simulink model "c_station_v3"  (R2019a)
settings: Solver=VariableStepAuto  StartTime=0.0  StopTime=345600  MaxStep=3600  RelTol=1e-3  AbsTol=1e-3  EnableMultiTasking=on
StopFcn:
  | displayGasParameters(gasPressures);
values from neighbouring files (symbols this model uses):
  conf = gasConfig()    [ColoradoGasModel.m]    (also in gas_v1.m)
  lineParm = [lineParm;add_line("Main 2",24,35,pNom)]    [compressorTest.m]    (also in experiment1.m = [lineParm;add_line("Main 2",24,50,pNom)]; experiment2.m = [lineParm;add_line("Main 3",24,35,pNom)]; experiment3.m = [lineParm;add_line("Aux 3",36,100,pNom)]; experiments12.m)
  loadControlFlag = "on"    [gas_v1.m]
  loadParm = [loadParm; add_load("PP2",pwr,pNom,pCut, stopTime)]    [compressorTest.m]    (also in experiment1.m; experiment2.m; experiment3.m = [loadParm; add_load("PP2",pwr,pNom,pCut,stopTime)]; experiments12.m)
  valveControlFlag = "on"    [ColoradoGasModel.m]    (also in gas_v1.m)
undefined symbols (not defined in the file or in its folder): f, valveParm
libraries: gasLibrary x27, fl_lib x14, nesl_utility x9, instrumentlib x4, SimscapeFluids_lib x1
(part 3 of 3)

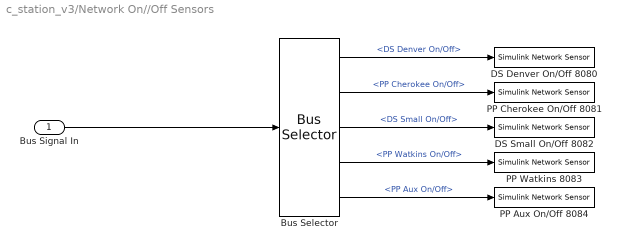
== system c_station_v3/Network On//Off Sensors ==
  Bus Signal In : Inport
  Bus Selector : BusSelector  OutputSignals=DS Denver On/Off,PP Cherokee On/Off,DS Small On/Off,PP Watkins On/Off,PP Aux On/Off
  DS Denver On/Off 8080 : gasLibrary/Simulink Network Sensor  Port=8080
  DS Small On/Off 8082 : gasLibrary/Simulink Network Sensor  Port=8082
  PP Aux On/Off 8084 : gasLibrary/Simulink Network Sensor  Port=8084
  PP Cherokee On/Off 8081 : gasLibrary/Simulink Network Sensor  Port=8081
  PP Watkins 8083 : gasLibrary/Simulink Network Sensor  Port=8083
  wires:
  Bus Selector/1 -> DS Denver On/Off 8080/1  "<DS Denver On/Off>"
  Bus Signal In/1 -> Bus Selector/1
  Bus Selector/2 -> PP Cherokee On/Off 8081/1  "<PP Cherokee On/Off>"
  Bus Selector/4 -> PP Watkins 8083/1  "<PP Watkins On/Off>"
  Bus Selector/5 -> PP Aux On/Off 8084/1  "<PP Aux On/Off>"
  Bus Selector/3 -> DS Small On/Off 8082/1  "<DS Small On/Off>"

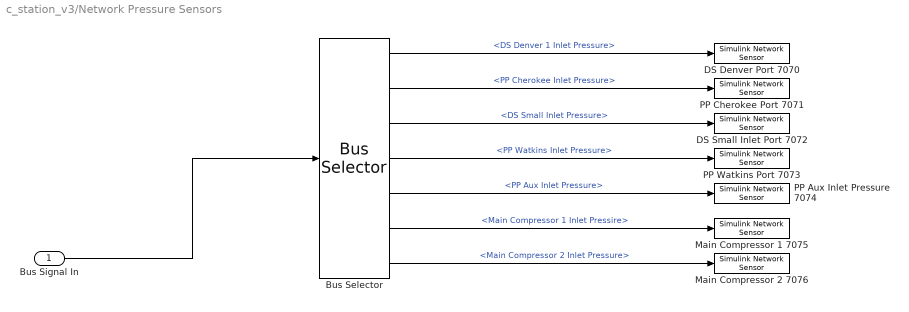
== system c_station_v3/Network Pressure Sensors ==
  Bus Signal In : Inport
  Bus Selector : BusSelector  OutputSignals=DS Denver 1 Inlet Pressure,PP Cherokee Inlet Pressure,DS Small Inlet Pressure,PP Watkins Inlet Pressure,PP Aux Inlet Pressure,Main Compressor 1 Inlet Pressire,Main Compressor 2 Inlet Pressure
  DS Denver Port 7070 : gasLibrary/Simulink Network Sensor  Port=7070
  DS Small Inlet Port 7072 : gasLibrary/Simulink Network Sensor  Port=7072
  Main Compressor 1 7075 : gasLibrary/Simulink Network Sensor  Port=7075
  Main Compressor 2 7076 : gasLibrary/Simulink Network Sensor  Port=7076
  PP Aux Inlet Pressure 7074 : gasLibrary/Simulink Network Sensor  Port=7074
  PP Cherokee Port 7071 : gasLibrary/Simulink Network Sensor  Port=7071
  PP Watkins Port 7073 : gasLibrary/Simulink Network Sensor  Port=7073
  wires:
  Bus Selector/4 -> PP Watkins Port 7073/1  "<PP Watkins Inlet Pressure>"
  Bus Signal In/1 -> Bus Selector/1
  Bus Selector/2 -> PP Cherokee Port 7071/1  "<PP Cherokee Inlet Pressure>"
  Bus Selector/3 -> DS Small Inlet Port 7072/1  "<DS Small Inlet Pressure>"
  Bus Selector/1 -> DS Denver Port 7070/1  "<DS Denver 1 Inlet Pressure>"
  Bus Selector/6 -> Main Compressor 1 7075/1  "<Main Compressor 1 Inlet Pressire>"
  Bus Selector/7 -> Main Compressor 2 7076/1  "<Main Compressor 2 Inlet Pressure>"
  Bus Selector/5 -> PP Aux Inlet Pressure 7074/1  "<PP Aux Inlet Pressure>"

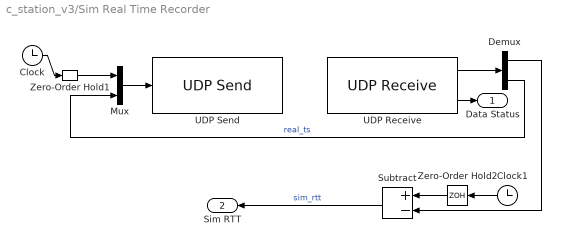
== system c_station_v3/Sim Real Time Recorder ==
  Clock : Clock
  Clock1 : Clock
  Demux : Demux  Outputs=2
  Mux : Mux  Inputs=2
  Subtract : Sum  Inputs=+-
  UDP Receive : instrumentlib/UDP Receive  Priority=2  Host=localhost  Port=5001  LocalPort=6065  EnablePortSharing=off  GetLatestData=off  DataSize="[2  1]"  DataType=double  ASCIIFormatting=%f,  Terminator=LF  ByteOrder=BigEndian  EnableBlockingMode=off  Timeout=50  SampleTime=60  LocalAddress=localhost
      settings: SourceProductName=Instrument Control Toolbox
  UDP Send : instrumentlib/UDP Send  Priority=1  Host=localhost  Port=6068  LocalPort=-1  EnablePortSharing=off  ByteOrder=BigEndian  OutputDatagramPacketSize=24  EnableBlockingMode=on  LocalAddress=0.0.0.0
      settings: SourceProductName=Instrument Control Toolbox
  Zero-Order Hold1 : ZeroOrderHold  SampleTime=60
  Zero-Order Hold2 : ZeroOrderHold  SampleTime=60
  Data Status : Outport
  Sim RTT : Outport  Port=2
  wires:
  Clock1/1 -> Zero-Order Hold2/1
  Clock/1 -> Zero-Order Hold1/1
  Demux/1 -> Subtract/2
  UDP Receive/1 -> Demux/1
  Demux/2 -> Mux/2  "real_ts"
  UDP Receive/2 -> Data Status/1
  Mux/1 -> UDP Send/1
  Zero-Order Hold2/1 -> Subtract/1
  Zero-Order Hold1/1 -> Mux/1
  Subtract/1 -> Sim RTT/1  "sim_rtt"

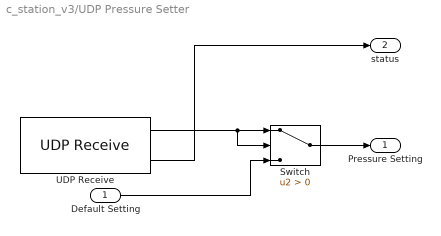
== system c_station_v3/UDP Pressure Setter ==
  Default Setting : Inport
  Switch : Switch  Criteria=u2 > Threshold
  UDP Receive : instrumentlib/UDP Receive  Host=localhost  Port=5000  LocalPort=LocalPort  EnablePortSharing=off  GetLatestData=on  DataSize=[1 1]  DataType=double  ASCIIFormatting=%f,  Terminator=LF  ByteOrder=BigEndian  EnableBlockingMode=off  Timeout=10  SampleTime=300  LocalAddress=localhost
      settings: SourceProductName=Instrument Control Toolbox
  "Pressure Setting " : Outport
  status : Outport  Port=2
  wires:
  UDP Receive/2 -> status/1
  UDP Receive/1 -> Switch/1, Switch/2
  Switch/1 -> "Pressure Setting "/1
  Default Setting/1 -> Switch/3

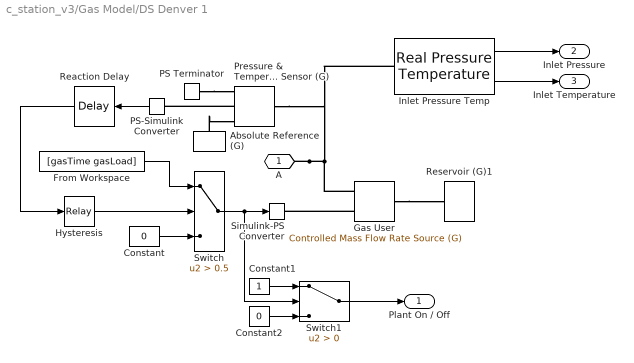
== system c_station_v3/Gas Model/DS Denver 1 ==
  Absolute Reference (G) : fl_lib/Gas/Elements/Absolute Reference (G)
      settings: SourceProductName=Simscape  SourceProductBaseCode=SS
  Constant : Constant  Value=0
  Constant1 : Constant
  Constant2 : Constant  Value=0
  From Workspace : FromWorkspace  VariableName=[gasTime gasLoad]  SampleTime=0  OutputAfterFinalValue=Holding final value
  Gas User : fl_lib/Gas/Sources/Controlled Mass Flow Rate Source (G)  power_spec=1  area_A=24^2*pi/4 in^2  area_B=20^2*pi/4 in^2  mdot_A_specify=on  mdot_A_priority=None  mdot_A=20 kg/s  mdot_A_nominal_specify=off  mdot_A_nominal_unit=kg/s  mdot_A_nominal_value=1
      settings: SourceProductName=Simscape  SourceProductBaseCode=SS
  Hysteresis : Relay  OnSwitchValue=pCutoff*1.05  OffSwitchValue=pCutoff
  Inlet Pressure Temp : gasLibrary/Real Pressure Temperature  SystemSampleTime=-1
  PS Terminator : fl_lib/Physical Signals/Sinks/PS Terminator
      settings: SourceProductName=Simscape
  PS-Simulink Converter : nesl_utility/PS-Simulink Converter  PhysicalDomain=network_engine_domain  SubClassName=ps_output  LeftPortType=input  RightPortType=output  PseudoPeriodic=off  Frequencies=[]  Unit=psi  AffineConversion=off
  Pressure & Temperature Sensor (G) : fl_lib/Gas/Sensors/Pressure & Temperature Sensor (G)
      settings: SourceProductName=Simscape  SourceProductBaseCode=SS
  Reaction Delay : TransportDelay  DelayTime=60  InitialOutput=pNominal
  Reservoir (G)1 : fl_lib/Gas/Elements/Reservoir (G)  pressure_spec=2  reservoir_pressure=300 psi  reservoir_temperature=25 degC  area_A=pi*25^2/4 in^2
      settings: SourceProductName=Foundation Library
  Simulink-PS Converter : nesl_utility/Simulink-PS Converter  PhysicalDomain=network_engine_domain  SubClassName=ps_input  LeftPortType=input  RightPortType=output  PseudoPeriodic=off  Frequencies=[]  NoiseDistribution=none  NoiseParameters=[]  Unit=1  AffineConversion=off  FilteringAndDerivatives=provide  SimscapeFilterOrder=1  InputFilterTimeConstant=0.001  UdotUserProvided=0
  Switch : Switch  Criteria=u2 > Threshold  Threshold=0.5
  Switch1 : Switch  Criteria=u2 > Threshold
  A : PMIOPort  Side=Left
  Plant On / Off : Outport
  Inlet Pressure : Outport  Port=2
  Inlet Temperature : Outport  Port=3
  wires:
  Inlet Pressure Temp/2 -> Inlet Temperature/1
  Inlet Pressure Temp/1 -> Inlet Pressure/1
  Constant1/1 -> Switch1/1
  Switch1/1 -> Plant On / Off/1
  Constant2/1 -> Switch1/3
  Switch/1 -> Simulink-PS Converter/1, Switch1/2
  Hysteresis/1 -> Switch/2
  Constant/1 -> Switch/3
  PS-Simulink Converter/1 -> Reaction Delay/1
  Reaction Delay/1 -> Hysteresis/1
  From Workspace/1 -> Switch/1
  connections:
  Pressure & Temperature Sensor (G)/RConn2 -- PS-Simulink Converter/LConn1
  Absolute Reference (G)/LConn1 -- Pressure & Temperature Sensor (G)/RConn1
  PS Terminator/LConn1 -- Pressure & Temperature Sensor (G)/RConn3
  Gas User/LConn2 -- Simulink-PS Converter/RConn1
  A/RConn1 -- Pressure & Temperature Sensor (G)/LConn1 -- Inlet Pressure Temp/LConn1 -- Gas User/LConn1
  Gas User/RConn1 -- Reservoir (G)1/LConn1

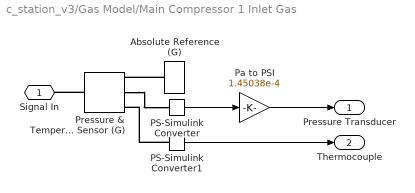
== system c_station_v3/Gas Model/Main Compressor 1 Inlet Gas ==
  Absolute Reference (G) : fl_lib/Gas/Elements/Absolute Reference (G)
      settings: SourceProductName=Simscape  SourceProductBaseCode=SS
  PS-Simulink Converter : nesl_utility/PS-Simulink Converter  PhysicalDomain=network_engine_domain  SubClassName=ps_output  LeftPortType=input  RightPortType=output  PseudoPeriodic=off  Frequencies=[]  Unit=1  AffineConversion=off
  PS-Simulink Converter1 : nesl_utility/PS-Simulink Converter  PhysicalDomain=network_engine_domain  SubClassName=ps_output  LeftPortType=input  RightPortType=output  PseudoPeriodic=off  Frequencies=[]  Unit=1  AffineConversion=off
  Pa to PSI : Gain  Gain=1.45038e-4
  Pressure & Temperature Sensor (G) : fl_lib/Gas/Sensors/Pressure & Temperature Sensor (G)
      settings: SourceProductName=Simscape  SourceProductBaseCode=SS
  Signal In : PMIOPort  Side=Left
  Pressure Transducer : Outport
  Thermocouple : Outport  Port=2
  wires:
  PS-Simulink Converter/1 -> Pa to PSI/1
  PS-Simulink Converter1/1 -> Thermocouple/1
  Pa to PSI/1 -> Pressure Transducer/1
  connections:
  Pressure & Temperature Sensor (G)/LConn1 -- Signal In/RConn1
  Absolute Reference (G)/LConn1 -- Pressure & Temperature Sensor (G)/RConn1
  PS-Simulink Converter1/LConn1 -- Pressure & Temperature Sensor (G)/RConn3
  Pressure & Temperature Sensor (G)/RConn2 -- PS-Simulink Converter/LConn1

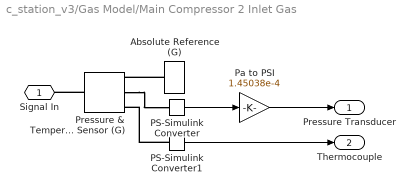
== system c_station_v3/Gas Model/Main Compressor 2 Inlet Gas ==
  Absolute Reference (G) : fl_lib/Gas/Elements/Absolute Reference (G)
      settings: SourceProductName=Simscape  SourceProductBaseCode=SS
  PS-Simulink Converter : nesl_utility/PS-Simulink Converter  PhysicalDomain=network_engine_domain  SubClassName=ps_output  LeftPortType=input  RightPortType=output  PseudoPeriodic=off  Frequencies=[]  Unit=1  AffineConversion=off
  PS-Simulink Converter1 : nesl_utility/PS-Simulink Converter  PhysicalDomain=network_engine_domain  SubClassName=ps_output  LeftPortType=input  RightPortType=output  PseudoPeriodic=off  Frequencies=[]  Unit=1  AffineConversion=off
  Pa to PSI : Gain  Gain=1.45038e-4
  Pressure & Temperature Sensor (G) : fl_lib/Gas/Sensors/Pressure & Temperature Sensor (G)
      settings: SourceProductName=Simscape  SourceProductBaseCode=SS
  Signal In : PMIOPort  Side=Left
  Pressure Transducer : Outport
  Thermocouple : Outport  Port=2
  wires:
  PS-Simulink Converter/1 -> Pa to PSI/1
  PS-Simulink Converter1/1 -> Thermocouple/1
  Pa to PSI/1 -> Pressure Transducer/1
  connections:
  Pressure & Temperature Sensor (G)/LConn1 -- Signal In/RConn1
  Absolute Reference (G)/LConn1 -- Pressure & Temperature Sensor (G)/RConn1
  PS-Simulink Converter1/LConn1 -- Pressure & Temperature Sensor (G)/RConn3
  Pressure & Temperature Sensor (G)/RConn2 -- PS-Simulink Converter/LConn1

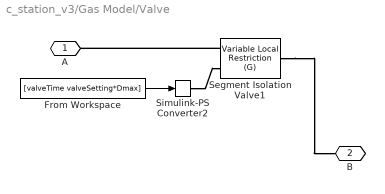
== system c_station_v3/Gas Model/Valve ==
  From Workspace : FromWorkspace  VariableName=[valveTime valveSetting*Dmax]  SampleTime=0  OutputAfterFinalValue=Holding final value
  Segment Isolation Valve1 : fl_lib/Gas/Elements/Variable Local Restriction (G)  min_area=1e-4 in^2  max_area=pi*(Dmax-1)^2/4 in^2  area=pi*D^2/4 in^2  Cd=0.64  B_lam=0.999  mdot_A_specify=off  mdot_A_priority=None  mdot_A=1e-6 kg/s  mdot_A_nominal_specify=off  mdot_A_nominal_unit=kg/s  mdot_A_nominal_value=1
      settings: SourceProductName=Simscape  SourceProductBaseCode=SS
  Simulink-PS Converter2 : nesl_utility/Simulink-PS Converter  PhysicalDomain=network_engine_domain  SubClassName=ps_input  LeftPortType=input  RightPortType=output  PseudoPeriodic=off  Frequencies=[]  NoiseDistribution=none  NoiseParameters=[]  Unit=in^2  AffineConversion=off  FilteringAndDerivatives=provide  SimscapeFilterOrder=1  InputFilterTimeConstant=0.001  UdotUserProvided=0
  A : PMIOPort  Side=Left
  B : PMIOPort  Port=2  Side=Right
  wires:
  From Workspace/1 -> Simulink-PS Converter2/1
  connections:
  Simulink-PS Converter2/RConn1 -- Segment Isolation Valve1/LConn2
  Segment Isolation Valve1/LConn1 -- A/RConn1
  Segment Isolation Valve1/RConn1 -- B/RConn1

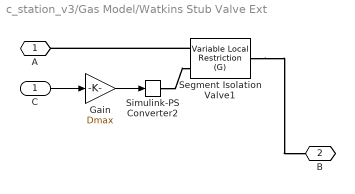
== system c_station_v3/Gas Model/Watkins Stub Valve Ext ==
  C : Inport
  Gain : Gain  Gain=Dmax
  Segment Isolation Valve1 : fl_lib/Gas/Elements/Variable Local Restriction (G)  min_area=1e-4 in^2  max_area=pi*(Dmax-1)^2/4 in^2  area=pi*D^2/4 in^2  Cd=0.64  B_lam=0.999  mdot_A_specify=off  mdot_A_priority=None  mdot_A=1e-6 kg/s  mdot_A_nominal_specify=off  mdot_A_nominal_unit=kg/s  mdot_A_nominal_value=1
      settings: SourceProductName=Simscape  SourceProductBaseCode=SS
  Simulink-PS Converter2 : nesl_utility/Simulink-PS Converter  PhysicalDomain=network_engine_domain  SubClassName=ps_input  LeftPortType=input  RightPortType=output  PseudoPeriodic=off  Frequencies=[]  NoiseDistribution=none  NoiseParameters=[]  Unit=in^2  AffineConversion=off  FilteringAndDerivatives=provide  SimscapeFilterOrder=1  InputFilterTimeConstant=0.001  UdotUserProvided=0
  A : PMIOPort  Side=Left
  B : PMIOPort  Port=2  Side=Right
  wires:
  C/1 -> Gain/1
  Gain/1 -> Simulink-PS Converter2/1
  connections:
  Segment Isolation Valve1/RConn1 -- B/RConn1
  Segment Isolation Valve1/LConn1 -- A/RConn1
  Simulink-PS Converter2/RConn1 -- Segment Isolation Valve1/LConn2

== matlab function c_station_v3/Gas Model/MATLAB Function ==
  data: loadOutputs output; loadStates input; currentLoad parameter
function loadOutputs  = fcn(loadStates, currentLoad)

loadsUp = 0;
for i = loadStates
    if i == 0
        loadsUp = loadsUp + 1;
    end
end

loadDist = currentLoad / loadsUp;
loadOutputs = loadDist;
